simulink model "purePursuitController"  (R2022b)
settings: Solver=VariableStepAuto  StartTime=0.0  StopTime=inf  RelTol=1e-3
values from neighbouring files (symbols this model uses):
  xRef = xRef2s    [dataVisualizer.m]    (also in tunningPP.m)
  yRef = yRef2s    [dataVisualizer.m]    (also in tunningPP.m)
undefined symbols (not defined in the file or in its folder): Angular, L, ld, Linear
libraries: robotlib x3, robotalgslib x1
settings Model: Creator=kisho  LastModifiedBy=kishor
settings DebuggingCC: UnconnectedInputMsg=warning  UnconnectedOutputMsg=warning  UnconnectedLineMsg=warning
settings ModelReferenceCC: EnableRefExpFcnMdlSchedulingChecks=on
settings RTWCC: DLArmComputeVersion=19.05

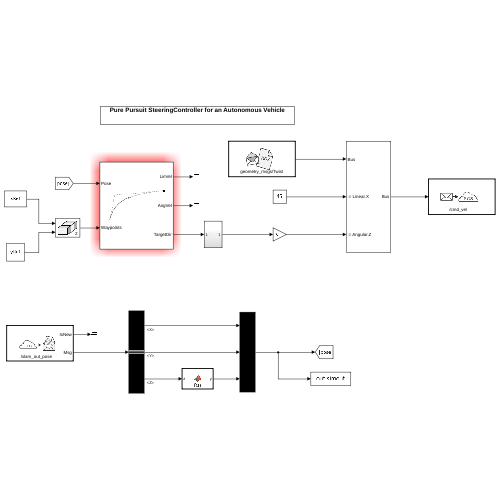
[thumbnail: Simulink's stored preview of the top-level diagram]
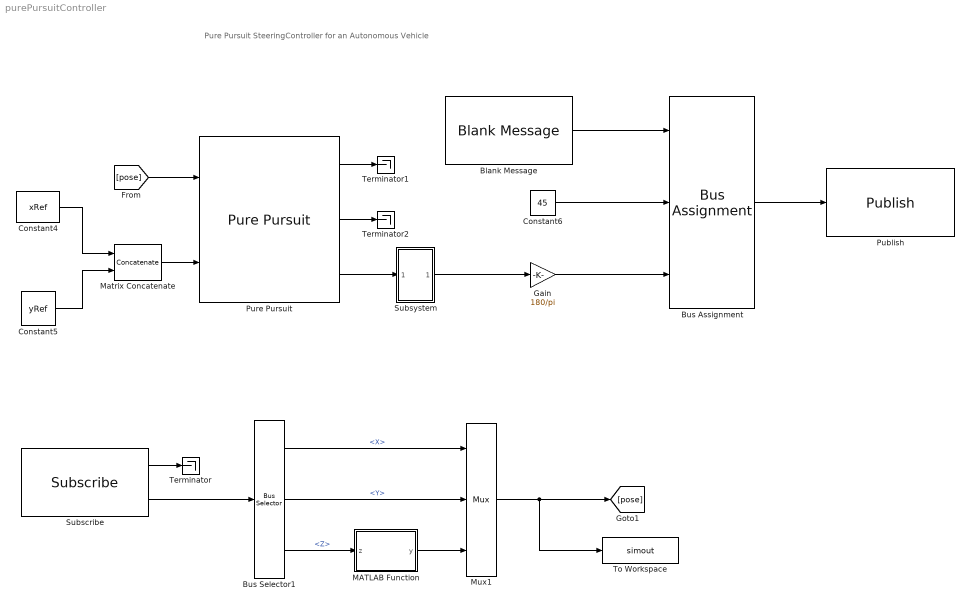
== system purePursuitController ==
  note: Pure Pursuit SteeringController for an Autonomous Vehicle
  Blank Message : robotlib/Blank Message  messageClass=Message  entityType=geometry_msgs/Twist  messageType=geometry_msgs/Twist  SampleTime=0.05  legacyBusStruct=off
      settings: LibrarySourceBlock=roslib/ROS/Blank Message
  Bus Assignment : BusAssignment  AssignedSignals=Linear.X,Angular.Z
  Bus Selector1 : BusSelector  OutputSignals=Pose.Position.X,Pose.Position.Y,Pose.Orientation.Z
  Constant4 : Constant  Value=xRef
  Constant5 : Constant  Value=yRef
  Constant6 : Constant  Value=45
  Gain : Gain  Gain=180/pi
  MATLAB Function : MATLAB Function  TreatAsAtomicUnit=on
  Matrix Concatenate : Concatenate  Mode=Multidimensional array  ConcatenateDimension=2
  Mux1 : Mux  Inputs=3
  Publish : robotlib/Publish  topicSource=Specify your own  topic=/cmd_vel  messageType=geometry_msgs/Twist  legacyBusStruct=off  messageQueueLength=1
      settings: LibrarySourceBlock=roslib/ROS/Publish
  Pure Pursuit : robotalgslib/Pure Pursuit  DesiredLinearVelocity=0.5  MaxAngularVelocity=1.0  LookaheadDistance=ld  TargetDirPort=on  SimulateUsing=Code generation
  Subscribe : robotlib/Subscribe  topicSource=Specify your own  topic=/slam_out_pose  messageType=geometry_msgs/PoseStamped  SampleTime=0.05  legacyBusStruct=off  messageQueueLength=1
      settings: LibrarySourceBlock=roslib/ROS/Subscribe
  Subsystem : Subsystem
  Terminator : Terminator
  Terminator1 : Terminator
  Terminator2 : Terminator
  To Workspace : ToWorkspace  VariableName=simout  SaveFormat=Timeseries  SampleTime=-1
  wires:
  Constant4/1 -> Matrix Concatenate/1
  Constant5/1 -> Matrix Concatenate/2
  Matrix Concatenate/1 -> Pure Pursuit/2
  [pose] -> Pure Pursuit/1
  Subsystem/1(Out1) -> Gain/1
  Blank Message/1 -> Bus Assignment/1
  Constant6/1 -> Bus Assignment/2
  Bus Assignment/1 -> Publish/1
  Subscribe/1 -> Terminator/1
  Subscribe/2 -> Bus Selector1/1
  Bus Selector1/1 -> Mux1/1  "<X>"
  Bus Selector1/2 -> Mux1/2  "<Y>"
  Bus Selector1/3 -> MATLAB Function/1(z)  "<Z>"
  Mux1/1 -> [pose], To Workspace/1
  Pure Pursuit/1 -> Terminator1/1
  Pure Pursuit/2 -> Terminator2/1
  MATLAB Function/1(y) -> Mux1/3
  Gain/1 -> Bus Assignment/3
  Pure Pursuit/3 -> Subsystem/1(In1)

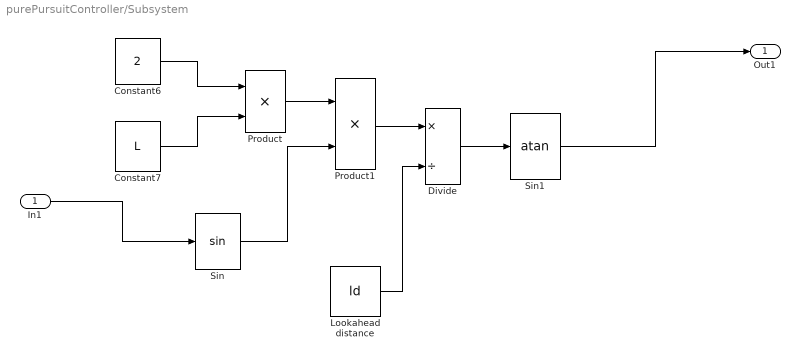
== system purePursuitController/Subsystem ==
  In1 : Inport
  Constant6 : Constant  Value=2
  Constant7 : Constant  Value=L
  Divide : Product  Inputs=*/
  Lookahead distance : Constant  Value=ld
  Product : Product
  Product1 : Product
  Sin : Trigonometry
  Sin1 : Trigonometry  Operator=atan
  Out1 : Outport
  wires:
  Divide/1 -> Sin1/1
  Lookahead distance/1 -> Divide/2
  Constant6/1 -> Product/1
  Product/1 -> Product1/1
  Product1/1 -> Divide/1
  In1/1 -> Sin/1
  Sin/1 -> Product1/2
  Constant7/1 -> Product/2
  Sin1/1 -> Out1/1

== matlab function purePursuitController/MATLAB Function ==
  data: z input; y output
function y = fcn(z)
z = z*pi;
if (z>0)
    y = z;
elseif (z<0)
    y = pi + (pi-z);
else
    y = z;
end
